simulink model "outrun_nn_breach"  (R2019a)
settings: Solver=ode5  StartTime=0.0  StopTime=20  FixedStep=.01  RelTol=1e-3  AbsTol=1e-6
model workspace (MATLAB code in the model file):
  | load sldemo_autotrans_data; %load initial conditions and other necessary data
undefined symbols (not defined in the file or in its folder): a_max, converter_data, downtab, emap, f_mu, Iei, panic_brake, speed_s0, T_h_delay, T_s_delay, TTC_inv_safe, TTC_inv_warning, uptab, vehicledata, warn_brake, x_p0, x_safe, x_warning
Description:
  | Modeling an Automatic Transmission Controller
  | 
  | In this example, Simulink(R) is used to model an automotive drivetrain. Stateflow(R)
  | enhances the Simulink model with its representation of the transmission
  | control logic. Simulink provides a powerful environment for the modeling and
  | simulation of dynamic systems and processes. In many systems, though,
  | supervisory functions like changing modes or invoking new gain schedules must
  | respond to events that may occur and conditions that develop over time. As a
  | result, the environment requires a language capable of managing these multiple
  | modes and developing conditions. In the following example, Stateflow
  | demonstrates its strength in this capacity by performing the function of gear
  | selection in an automatic transmission. This function is combined with the
  | drivetrain dynamics in a natural and intuitive manner by incorporating a
  | Stateflow block in the Simulink block diagram.
settings Model: DataTypeOverride=Double  MinMaxOverflowLogging=ForceOff  ExtModeTrigMode=oneshot  ExtModeArmWhenConnect=off  ExtModeAutoUpdateStatusClock=off  Creator=The MathWorks Inc.  LastModifiedBy=nikhil
settings SolverCC: AutoScaleAbsTol=off
settings DataIOCC: ExternalInput=[0 0 0 0]  LoadExternalInput=on  SaveFormat=StructureWithTime
settings OptimizationCC: BlockReduction=off  BooleanDataType=off  ExpressionDepthLimit=2147483647  InitFltsAndDblsToZero=on  LifeSpan=inf
settings DebuggingCC: SaveWithParameterizedLinksMsg=none  UnderspecifiedInitializationDetection=Classic  MergeDetectMultiDrivingBlocksExec=none  CheckExecutionContextPreStartOutputMsg=on  CheckExecutionContextRuntimeOutputMsg=on  SignalResolutionControl=TryResolveAllWithWarning  MultiTaskDSMMsg=warning  MultiTaskCondExecSysMsg=none  SigSpecEnsureSampleTimeMsg=none  IntegerOverflowMsg=none  FcnCallInpInsideContextMsg=warning  StateNameClashWarn=warning  SFUnexpectedBacktrackingDiag=warning  SFNoUnconditionalDefaultTransitionDiag=warning  SFExecutionAtInitializationDiag=none  IntegerSaturationMsg=none  ArithmeticOperatorsInVariantConditions=warning
settings HardwareCC: ProdBitPerPointer=32  ProdBitPerSizeT=32  ProdBitPerPtrDiffT=32  ProdLargestAtomicFloat=None  ProdIntDivRoundTo=Undefined  ProdEndianess=Unspecified  ProdWordSize=32  ProdHWDeviceType=32-bit Generic
settings ModelReferenceCC: PropagateSignalLabelsOutOfModel=off
settings SFSimCC: SFSimEcho=off  SimUseLocalCustomCode=off
settings RTWCC: RTWUseLocalCustomCode=off
settings CodeAppCC: StateflowObjectComments=on
settings GRTTargetCC: TargetFcnLib=ansi_tfl_tmw.mat  TargetLangStandard=C89/C90 (ANSI)  GeneratePreprocessorConditionals=Disable all  CombineOutputUpdateFcns=off  GRTInterface=on
settings ConfigComp: CovMetricSettings=dcmtr  CovHtmlReporting=on  CovSaveCumulativeToWorkspaceVar=on  CovSaveSingleToWorkspaceVar=on  CovExternalEMLEnable=off  CovSFcnEnable=off

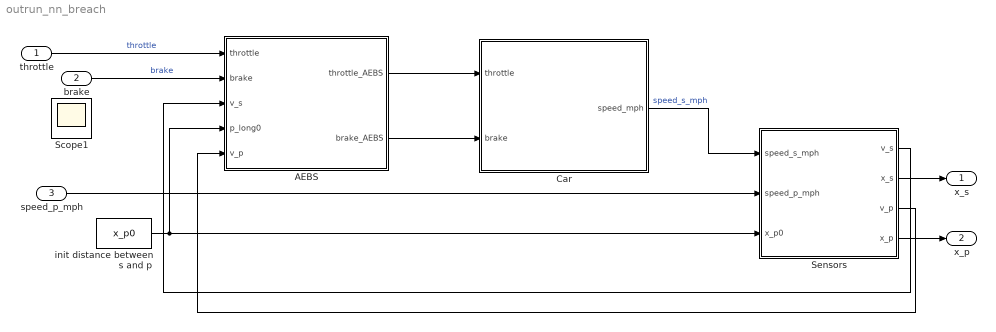
== system outrun_nn_breach ==
  throttle : Inport  Interpolate=off
  brake : Inport  Port=2  Interpolate=off
  speed_p_mph : Inport  Port=3  Interpolate=off
  AEBS : Subsystem
  Car : Subsystem
  Sensors : Subsystem
  init distance between s and p : Constant  Value=x_p0
  x_s : Outport
  x_p : Outport  Port=2
  Scope1 : Scope
  wires:
  throttle/1 -> AEBS/1(throttle)  "throttle"
  brake/1 -> AEBS/2(brake)  "brake"
  AEBS/1(throttle_AEBS) -> Car/1(throttle)
  AEBS/2(brake_AEBS) -> Car/2(brake)
  init distance between s and p/1 -> AEBS/4(p_long0), Sensors/3(x_p0)
  Car/1(speed_mph) -> Sensors/1(speed_s_mph)  "speed_s_mph"
  Sensors/1(v_s) -> AEBS/3(v_s)
  Sensors/2(x_s) -> x_s/1
  Sensors/3(v_p) -> AEBS/5(v_p)
  Sensors/4(x_p) -> x_p/1
  speed_p_mph/1 -> Sensors/2(speed_p_mph)

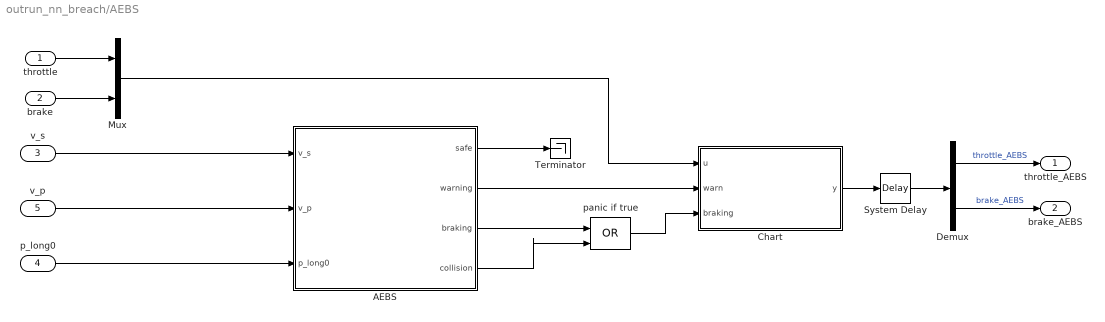
== system outrun_nn_breach/AEBS ==
  throttle : Inport
  brake : Inport  Port=2
  v_s : Inport  Port=3
  p_long0 : Inport  Port=4
  v_p : Inport  Port=5
  AEBS : Subsystem
  Chart : Stateflow chart  TreatAsAtomicUnit=on
  Demux : Demux  Outputs=2
  Mux : Mux  Inputs=2
  "System Delay " : TransportDelay  DelayTime=T_s_delay
  Terminator : Terminator
  panic if true : Logic  Operator=OR  IconShape=distinctive  AllPortsSameDT=off  OutDataTypeStr=boolean
  throttle_AEBS : Outport
  brake_AEBS : Outport  Port=2
  wires:
  Demux/1 -> throttle_AEBS/1  "throttle_AEBS"
  panic if true/1 -> Chart/3(braking)
  Mux/1 -> Chart/1(u)
  brake/1 -> Mux/2
  v_s/1 -> AEBS/1(v_s)
  "System Delay "/1 -> Demux/1
  Chart/1(y) -> "System Delay "/1
  AEBS/2(warning) -> Chart/2(warn)
  throttle/1 -> Mux/1
  v_p/1 -> AEBS/2(v_p)
  p_long0/1 -> AEBS/3(p_long0)
  Demux/2 -> brake_AEBS/1  "brake_AEBS"
  AEBS/4(collision) -> panic if true/2
  AEBS/3(braking) -> panic if true/1
  AEBS/1(safe) -> Terminator/1

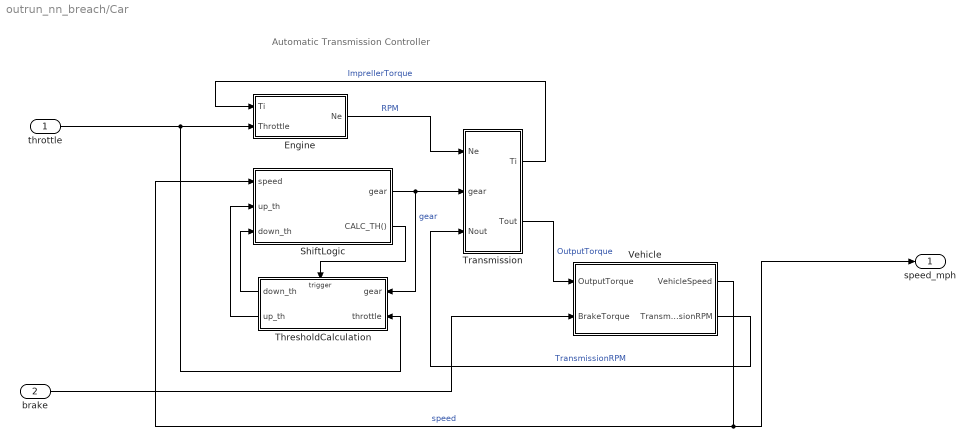
== system outrun_nn_breach/Car ==
  note: Automatic Transmission Controller
  throttle : Inport  Interpolate=off
  brake : Inport  Port=2  Interpolate=off
  Engine : Subsystem
  ShiftLogic : Stateflow chart  TreatAsAtomicUnit=on
  ThresholdCalculation : Subsystem  TreatAsAtomicUnit=on
  Transmission : Subsystem
  Vehicle : Subsystem  mask(vehicle model){Rfd=vehicledata(1), rload0=vehicledata(2), rload2=vehicledata(3), Rw=vehicledata(4), Iv=vehicledata(5), N20=speed_s0/0.022106666666667}
      mask prompts: Rfd "final drive ratio"; rload0 "drag friction at wheels"; rload2 "aerodynamic drag"; Rw "wheel radius"; Iv "vehicle inertia"; N20 "initial transmission output speed"
      mask help: vehicle dynamics: torque input from trans., outputs are input speed (transmission output) and vehicle speed
      mask Display: image(imread([matlabroot,'/toolbox/simulink/simdemos/automotive/html/NSX_3Colors.jpg']))
  speed_mph : Outport
  wires:
  ThresholdCalculation/1(down_th) -> ShiftLogic/3(down_th)
  ThresholdCalculation/2(up_th) -> ShiftLogic/2(up_th)
  throttle/1 -> Engine/2(Throttle), ThresholdCalculation/2(throttle)
  ShiftLogic/1(gear) -> Transmission/2(gear), ThresholdCalculation/1(gear)  "gear"
  ShiftLogic/2(CALC_TH()) -> ThresholdCalculation/Trigger
  Vehicle/1(VehicleSpeed) -> speed_mph/1, ShiftLogic/1(speed)  "speed"
  Transmission/2(Tout) -> Vehicle/1(OutputTorque)  "OutputTorque"
  brake/1 -> Vehicle/2(BrakeTorque)
  Transmission/1(Ti) -> Engine/1(Ti)  "ImprellerTorque"
  Vehicle/2(TransmissionRPM) -> Transmission/3(Nout)  "TransmissionRPM"
  Engine/1(Ne) -> Transmission/1(Ne)  "RPM"

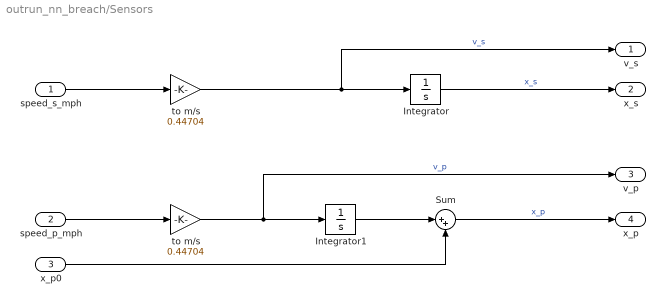
== system outrun_nn_breach/Sensors ==
  speed_s_mph : Inport
  speed_p_mph : Inport  Port=2
  x_p0 : Inport  Port=3
  " to m/s" : Gain  Gain=0.44704
  Integrator : Integrator
  Integrator1 : Integrator
  Sum : Sum  Inputs=|++
  to m/s : Gain  Gain=0.44704
  v_s : Outport
  x_s : Outport  Port=2
  v_p : Outport  Port=3
  x_p : Outport  Port=4
  wires:
  to m/s/1 -> v_s/1, Integrator/1  "v_s"
  " to m/s"/1 -> v_p/1, Integrator1/1  "v_p"
  Integrator/1 -> x_s/1  "x_s"
  speed_s_mph/1 -> to m/s/1
  Sum/1 -> x_p/1  "x_p"
  Integrator1/1 -> Sum/1
  speed_p_mph/1 -> " to m/s"/1
  x_p0/1 -> Sum/2

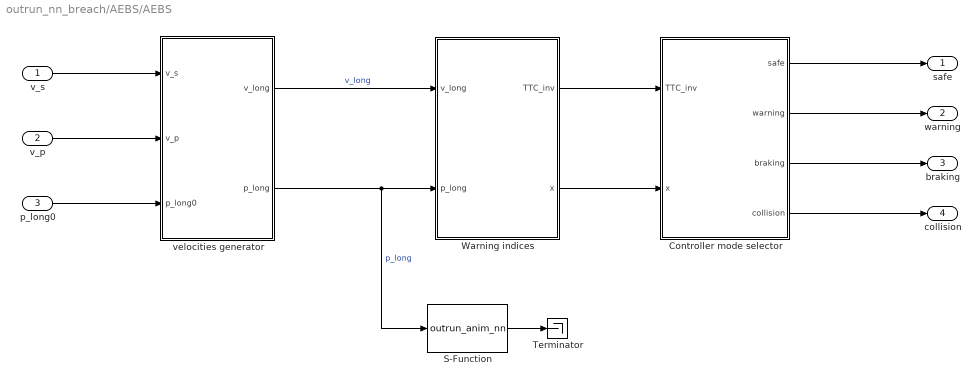
== system outrun_nn_breach/AEBS/AEBS ==
  v_s : Inport
  v_p : Inport  Port=2
  p_long0 : Inport  Port=3
  Controller mode selector : Subsystem
  S-Function : M-S-Function  FunctionName=outrun_anim_nn  Parameters=0
  Terminator : Terminator
  Warning indices : Subsystem
  velocities generator : Subsystem
  safe : Outport
  warning : Outport  Port=2
  braking : Outport  Port=3
  collision : Outport  Port=4
  wires:
  velocities generator/1(v_long) -> Warning indices/1(v_long)  "v_long"
  velocities generator/2(p_long) -> S-Function/1, Warning indices/2(p_long)  "p_long"
  p_long0/1 -> velocities generator/3(p_long0)
  v_p/1 -> velocities generator/2(v_p)
  v_s/1 -> velocities generator/1(v_s)
  Warning indices/1(TTC_inv) -> Controller mode selector/1(TTC_inv)
  Warning indices/2(x) -> Controller mode selector/2(x)
  Controller mode selector/1(safe) -> safe/1
  Controller mode selector/2(warning) -> warning/1
  Controller mode selector/3(braking) -> braking/1
  Controller mode selector/4(collision) -> collision/1
  S-Function/1 -> Terminator/1

== system outrun_nn_breach/Car/Engine ==
  note: Engine
  Ti : Inport
  Throttle : Inport  Port=2
  EngineTorque : Lookup2D  RowIndex=thvec  ColumnIndex=nevec  Table=emap  InputSameDT=on
  Integrator : Integrator  InitialCondition=1000  LimitOutput=on  UpperSaturationLimit=6000  LowerSaturationLimit=600  ZeroCross=off
  Sum : Sum  Inputs=-+  SaturateOnIntegerOverflow=on  InputSameDT=on  OutDataTypeStr=Inherit: Same as first input
  engine + impeller inertia : Gain  Gain=1/Iei  SaturateOnIntegerOverflow=on  OutDataTypeStr=Inherit: Same as input  ParamDataTypeStr=Inherit: Same as input
  Ne : Outport  InitialOutput=0
  wires:
  Ti/1 -> Sum/1
  Throttle/1 -> EngineTorque/1
  Integrator/1 -> EngineTorque/2, Ne/1  "RPM"
  Sum/1 -> engine + impeller inertia/1
  engine + impeller inertia/1 -> Integrator/1
  EngineTorque/1 -> Sum/2

== system outrun_nn_breach/Car/ThresholdCalculation ==
  note: Threshold Calculation
  gear : Inport
  throttle : Inport  Port=2
  run : TriggerPort  TriggerType=function-call  VariantControl=Variant  ZeroCross=off
  interp_down : Lookup2D  RowIndex=downth  ColumnIndex=[1:4]  Table=downtab  OutDataTypeStr=double
      settings: LockScale=on
  interp_up : Lookup2D  RowIndex=upth  ColumnIndex=[1:4]  Table=uptab  OutDataTypeStr=double
      settings: LockScale=on
  down_th : Outport
  up_th : Outport  Port=2
  wires:
  interp_up/1 -> up_th/1
  interp_down/1 -> down_th/1
  throttle/1 -> interp_up/1, interp_down/1
  gear/1 -> interp_up/2, interp_down/2

== system outrun_nn_breach/Car/Transmission ==
  note: Transmission
  Ne : Inport
  gear : Inport  Port=2
  Nout : Inport  Port=3
  TorqueConverter : Subsystem  mask(torque converter){speedratio=converter_data(:,1), Kfactor=converter_data(:,2), Torkratio=converter_data(:,3)}
      mask prompts: speedratio "speed ratio"; Kfactor "K factor"; Torkratio "torque ratio"
      mask help: torque converter
      mask Help: Torque converter input and output torques are computed as a function of the input and output speeds
      mask Display: plot([cos([90:10:450]*pi/180),.63*cos([90:10:450]*pi/180),.63*cos([90:10:240]*pi/180),cos([240:10:300]*pi/180),.63*cos([300]*pi/180)],[sin([90:10:450]*pi/180),.63*sin([90:10:450]*pi/180)+.1,.63*sin([90:10:240]*pi/180)+.1,sin([240:10:300]*pi/180),.63*sin([300]*pi/180)+.1])
  TransmissionRatio : Subsystem
  Ti : Outport  InitialOutput=0
  Tout : Outport  Port=2  InitialOutput=0
  wires:
  TransmissionRatio/1(Tout) -> Tout/1
  TorqueConverter/1(Ti) -> Ti/1
  Nout/1 -> TransmissionRatio/3(Nout)
  gear/1 -> TransmissionRatio/2(gear)
  Ne/1 -> TorqueConverter/1(Ne)
  TransmissionRatio/2(Nin) -> TorqueConverter/2(Nin)
  TorqueConverter/2(Tt) -> TransmissionRatio/1(Tin)  "turbine torque"

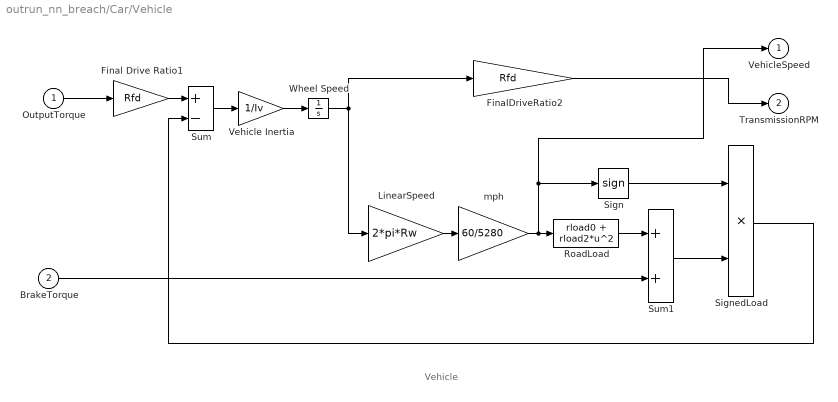
== system outrun_nn_breach/Car/Vehicle ==
  note: Vehicle
  OutputTorque : Inport
  BrakeTorque : Inport  Port=2
  Final Drive Ratio1 : Gain  Gain=Rfd  SaturateOnIntegerOverflow=on  OutDataTypeStr=Inherit: Same as input  ParamDataTypeStr=Inherit: Same as input
  FinalDriveRatio2 : Gain  Gain=Rfd  SaturateOnIntegerOverflow=on  OutDataTypeStr=Inherit: Same as input  ParamDataTypeStr=Inherit: Same as input
  LinearSpeed : Gain  Gain=2*pi*Rw  SaturateOnIntegerOverflow=on  OutDataTypeStr=Inherit: Same as input  ParamDataTypeStr=Inherit: Same as input
  RoadLoad : Fcn  Expr=rload0 + rload2*u^2
  Sign : Signum
  SignedLoad : Product  SaturateOnIntegerOverflow=on  InputSameDT=on  OutDataTypeStr=Inherit: Same as first input
  Sum : Sum  Inputs=+-  SaturateOnIntegerOverflow=on  InputSameDT=on  OutDataTypeStr=Inherit: Same as first input
  Sum1 : Sum  SaturateOnIntegerOverflow=on  InputSameDT=on  OutDataTypeStr=Inherit: Same as first input
  Vehicle Inertia : Gain  Gain=1/Iv  SaturateOnIntegerOverflow=on  OutDataTypeStr=Inherit: Same as input  ParamDataTypeStr=Inherit: Same as input
  Wheel Speed : Integrator  InitialCondition=N20/Rfd  ZeroCross=off
  mph : Gain  Gain=60/5280  SaturateOnIntegerOverflow=on  OutDataTypeStr=Inherit: Same as input  ParamDataTypeStr=Inherit: Same as input
  VehicleSpeed : Outport  InitialOutput=0
  TransmissionRPM : Outport  Port=2  InitialOutput=0
  wires:
  FinalDriveRatio2/1 -> TransmissionRPM/1
  BrakeTorque/1 -> Sum1/2
  Sum1/1 -> SignedLoad/2
  RoadLoad/1 -> Sum1/1
  Sign/1 -> SignedLoad/1
  SignedLoad/1 -> Sum/2
  OutputTorque/1 -> Final Drive Ratio1/1
  Vehicle Inertia/1 -> Wheel Speed/1
  Sum/1 -> Vehicle Inertia/1
  mph/1 -> VehicleSpeed/1, Sign/1, RoadLoad/1
  LinearSpeed/1 -> mph/1
  Wheel Speed/1 -> LinearSpeed/1, FinalDriveRatio2/1
  Final Drive Ratio1/1 -> Sum/1

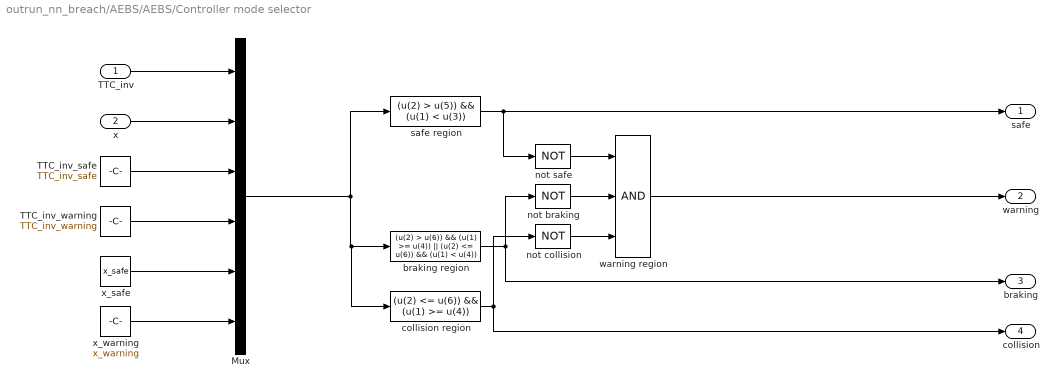
== system outrun_nn_breach/AEBS/AEBS/Controller mode selector ==
  TTC_inv : Inport
  x : Inport  Port=2
  Mux : Mux  Inputs=6
  TTC_inv_safe : Constant  Value=TTC_inv_safe
  TTC_inv_warning : Constant  Value=TTC_inv_warning
  braking region : Fcn  Expr=(u(2) > u(6)) && (u(1) >= u(4)) || (u(2) <= u(6)) && (u(1) < u(4))
  collision region : Fcn  Expr=(u(2) <= u(6)) && (u(1) >= u(4))
  not braking : Logic  Operator=NOT  Inputs=3  AllPortsSameDT=off  OutDataTypeStr=boolean
  not collision : Logic  Operator=NOT  Inputs=3  AllPortsSameDT=off  OutDataTypeStr=boolean
  not safe : Logic  Operator=NOT  Inputs=3  AllPortsSameDT=off  OutDataTypeStr=boolean
  safe region : Fcn  Expr=(u(2) > u(5)) && (u(1) < u(3))
  warning region : Logic  Inputs=3  AllPortsSameDT=off  OutDataTypeStr=boolean
  x_safe : Constant  Value=x_safe
  x_warning : Constant  Value=x_warning
  safe : Outport
  warning : Outport  Port=2
  braking : Outport  Port=3
  collision : Outport  Port=4
  wires:
  warning region/1 -> warning/1
  collision region/1 -> not collision/1, collision/1
  braking region/1 -> not braking/1, braking/1
  safe region/1 -> not safe/1, safe/1
  not collision/1 -> warning region/3
  not braking/1 -> warning region/2
  not safe/1 -> warning region/1
  Mux/1 -> braking region/1, collision region/1, safe region/1
  x_warning/1 -> Mux/6
  x_safe/1 -> Mux/5
  TTC_inv_warning/1 -> Mux/4
  TTC_inv_safe/1 -> Mux/3
  x/1 -> Mux/2
  TTC_inv/1 -> Mux/1

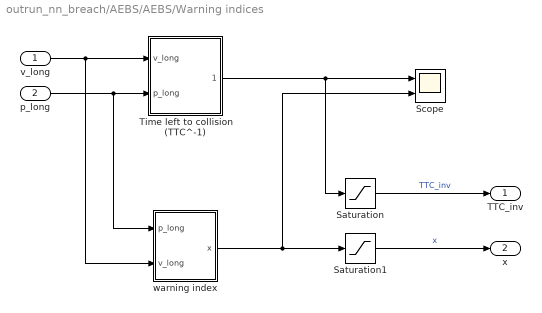
== system outrun_nn_breach/AEBS/AEBS/Warning indices ==
  v_long : Inport
  p_long : Inport  Port=2
  Saturation : Saturate  UpperLimit=10  LowerLimit=0
  Saturation1 : Saturate  UpperLimit=100  LowerLimit=-100
  Scope : Scope  NumInputPorts=2
  Time left to collision (TTC^-1) : Subsystem
  warning index : Subsystem
  TTC_inv : Outport
  x : Outport  Port=2
  wires:
  Time left to collision (TTC^-1)/1("TTC^-1 ") -> Saturation/1, Scope/1
  warning index/1("x ") -> Scope/2, Saturation1/1
  p_long/1 -> Time left to collision (TTC^-1)/2(p_long), warning index/1(p_long)
  v_long/1 -> Time left to collision (TTC^-1)/1(v_long), warning index/2(v_long)
  Saturation/1 -> TTC_inv/1  "TTC_inv"
  Saturation1/1 -> x/1  "x"

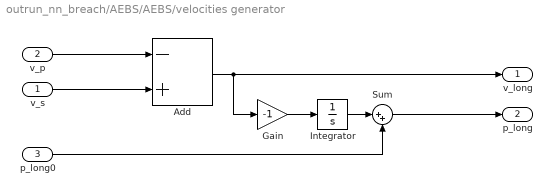
== system outrun_nn_breach/AEBS/AEBS/velocities generator ==
  v_s : Inport
  v_p : Inport  Port=2
  p_long0 : Inport  Port=3
  Add : Sum  Inputs=-+
  Gain : Gain  Gain=-1
  Integrator : Integrator
  Sum : Sum  Inputs=|++
  v_long : Outport
  p_long : Outport  Port=2
  wires:
  v_s/1 -> Add/2
  v_p/1 -> Add/1
  Add/1 -> Gain/1, v_long/1
  p_long0/1 -> Sum/2
  Integrator/1 -> Sum/1
  Sum/1 -> p_long/1
  Gain/1 -> Integrator/1

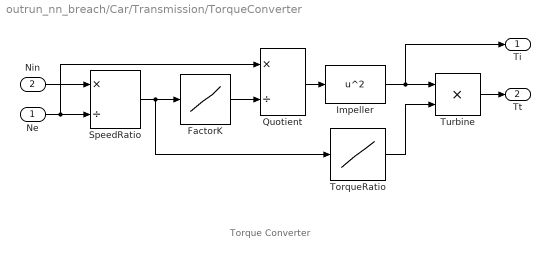
== system outrun_nn_breach/Car/Transmission/TorqueConverter ==
  note: Torque Converter
  Ne : Inport
  Nin : Inport  Port=2
  FactorK : Lookup  InputValues=speedratio  Table=Kfactor  SaturateOnIntegerOverflow=on
  Impeller : Fcn  Expr=u^2
  Quotient : Product  Inputs=*/  SaturateOnIntegerOverflow=on  InputSameDT=on  OutDataTypeStr=Inherit: Same as first input
  SpeedRatio : Product  Inputs=*/  SaturateOnIntegerOverflow=on  InputSameDT=on  OutDataTypeStr=Inherit: Same as first input
  TorqueRatio : Lookup  InputValues=speedratio  Table=Torkratio  SaturateOnIntegerOverflow=on
  Turbine : Product  SaturateOnIntegerOverflow=on  InputSameDT=on  OutDataTypeStr=Inherit: Same as first input
  Ti : Outport  InitialOutput=0
  Tt : Outport  Port=2  InitialOutput=0
  wires:
  TorqueRatio/1 -> Turbine/2
  Quotient/1 -> Impeller/1
  FactorK/1 -> Quotient/2
  SpeedRatio/1 -> TorqueRatio/1, FactorK/1
  Impeller/1 -> Turbine/1, Ti/1
  Turbine/1 -> Tt/1
  Ne/1 -> SpeedRatio/2, Quotient/1
  Nin/1 -> SpeedRatio/1

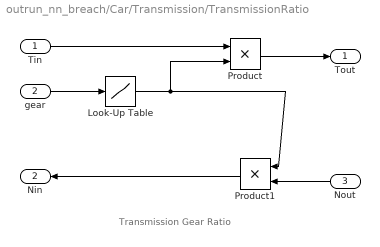
== system outrun_nn_breach/Car/Transmission/TransmissionRatio ==
  note: Transmission Gear Ratio
  Tin : Inport
  gear : Inport  Port=2
  Nout : Inport  Port=3
  Look-Up Table : Lookup  InputValues=[1 2 3 4]  Table=[2.393 1.450 1.000 0.677]  OutDataTypeStr=double  SaturateOnIntegerOverflow=on  LockScale=on
  Product : Product  SaturateOnIntegerOverflow=on  InputSameDT=on  OutDataTypeStr=Inherit: Same as first input
  Product1 : Product  SaturateOnIntegerOverflow=on  InputSameDT=on  OutDataTypeStr=Inherit: Same as first input
  Tout : Outport  InitialOutput=0
  Nin : Outport  Port=2  InitialOutput=0
  wires:
  Look-Up Table/1 -> Product1/1, Product/2
  Nout/1 -> Product1/2
  Product1/1 -> Nin/1
  Product/1 -> Tout/1
  Tin/1 -> Product/1
  gear/1 -> Look-Up Table/1

== system outrun_nn_breach/AEBS/AEBS/Warning indices/Time left to collision (TTC^-1) ==
  v_long : Inport
  p_long : Inport  Port=2
  Divide : Product  Inputs=*/
  "TTC^-1 " : Outport
  wires:
  Divide/1 -> "TTC^-1 "/1
  p_long/1 -> Divide/2
  v_long/1 -> Divide/1

== system outrun_nn_breach/AEBS/AEBS/Warning indices/warning index ==
  p_long : Inport
  v_long : Inport  Port=2
  Add : Sum  Inputs=+-
  Add1 : Sum  Inputs=+-
  Divide : Product  Inputs=*/
  "warning/braking critical distances " : Subsystem
  "x " : Outport
  wires:
  "warning/braking critical distances "/2(d_w) -> Add1/1  "d_w"
  Add/1 -> Divide/1
  v_long/1 -> "warning/braking critical distances "/1("v_long ")
  Divide/1 -> "x "/1  "x"
  p_long/1 -> Add/1
  Add1/1 -> Divide/2
  "warning/braking critical distances "/1(d_br) -> Add/2, Add1/2  "d_br"

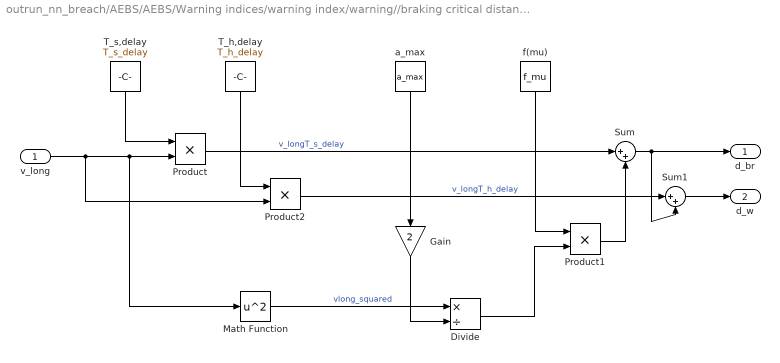
== system outrun_nn_breach/AEBS/AEBS/Warning indices/warning index/warning//braking critical distances  ==
  "v_long " : Inport
  Divide : Product  Inputs=*/
  Gain : Gain  Gain=2
  Math Function : Math  Operator=square  SaturateOnIntegerOverflow=on
  Product : Product
  Product1 : Product
  Product2 : Product
  Sum : Sum  Inputs=|++
  Sum1 : Sum  Inputs=|++
  T_h,delay : Constant  Value=T_h_delay
  T_s,delay : Constant  Value=T_s_delay
  a_max : Constant  Value=a_max
  f(mu) : Constant  Value=f_mu
  d_br : Outport
  d_w : Outport  Port=2
  wires:
  T_h,delay/1 -> Product2/1
  a_max/1 -> Gain/1
  Math Function/1 -> Divide/1  "vlong_squared"
  Sum/1 -> Sum1/2, d_br/1
  f(mu)/1 -> Product1/1
  Product1/1 -> Sum/2
  Sum1/1 -> d_w/1
  Product/1 -> Sum/1  "v_longT_s_delay"
  T_s,delay/1 -> Product/1
  Divide/1 -> Product1/2
  "v_long "/1 -> Product2/2, Math Function/1, Product/2
  Gain/1 -> Divide/2
  Product2/1 -> Sum1/1  "v_longT_h_delay"

== stateflow chart outrun_nn_breach/Car/ShiftLogic ==
  settings: updateMethod=DISCRETE  sampleTime=0.04
  state gear_state [parallel]
    settings: executionOrder=1
    state fourth
      entry:
      gear = 4;
    state third
      entry:
      gear = 3;
    state second
      entry:
      gear = 2;
    state first
      entry:
      gear = 1;
    (default) -> first
    second -> third [order 1] : UP
    first -> second : UP
    third -> fourth [order 1] : UP
    second -> first [order 2] : DOWN
    fourth -> third : DOWN
    third -> second [order 2] : DOWN
  state selection_state [parallel]
    during: CALC_TH;
    settings: executionOrder=2
    state steady_state
    state upshifting
    state downshifting
    (default) -> steady_state
    steady_state -> upshifting [order 1] : [speed > up_th]
    steady_state -> downshifting [order 2] : [speed < down_th]
    downshifting -> steady_state [order 2] : [speed > down_th]
    downshifting -> steady_state [order 1] : after(TWAIT,tick)
        | [speed <= down_th]
        | {gear_state.DOWN}
    upshifting -> steady_state [order 1] : after(TWAIT,tick)
        | [speed >= up_th]
        | {gear_state.UP}
    upshifting -> steady_state [order 2] : [speed < up_th]
  data: speed input double; gear output fixdt(0,8,5) [1..4]; TWAIT parameter fixdt(0,8,6); up_th input double; down_th input double
  events: DOWN local EITHER_EDGE_EVENT; UP local EITHER_EDGE_EVENT; CALC_TH output FUNCTION_CALL_EVENT

== stateflow chart outrun_nn_breach/AEBS/Chart ==
  state Warning
    entry:
    y=[0;warn_brake];
  state Panic
    entry: y=[0;panic_brake];
  state Normal
    entry: y=u;
  (default) -> Normal
  Normal -> Warning : [warn>0]
  Warning -> Panic [order 1] : [braking>0]
  Warning -> Normal [order 2] : [warn==0]
  data: u input; y output; warn input; braking input; panic_brake parameter; warn_brake parameter
